simulink model "Task14"  (R2019b)
settings: Solver=VariableStepAuto  StartTime=0.0  StopTime=10.0  RelTol=1e-3
settings Model: Creator=12393  LastModifiedBy=12393

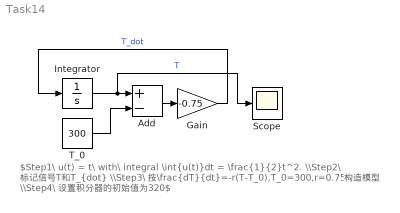
== system Task14 ==
  note: $Step1\ u(t) = t\ with\ integral \int{u(t)}dt = \frac{1}{2}t^2. \\Step2\ 标记信号T和T_{dot} \\Step3\ 按\frac{dT}{dt}=-r(T-T_0),T_0=300,r=0.75构造模型 \\Step4\ 设置积分器的初始值为320$
  Add : Sum  Inputs=+-
  Gain : Gain  Gain=-0.75
  Integrator : Integrator  InitialCondition=320
  Scope : Scope
  T_0 : Constant  Value=300
  wires:
  Gain/1 -> Integrator/1  "T_dot"
  Integrator/1 -> Scope/1, Add/1  "T"
  T_0/1 -> Add/2
  Add/1 -> Gain/1
